simulink model "gm_flash_led"  (R2026a)
settings: Solver=FixedStepDiscrete  StopTime=50
model workspace (MAT data in the model file):
  MAX_COUNT = 5000000
libraries: hdlsllib x2
settings Model: Creator=KoayXianCong  LastModifiedBy=KoayXianCong
settings OptimizationCC: ConditionallyExecuteInputs=off  InheritOutputTypeSmallerThanSingle=on
settings DebuggingCC: ArtificialAlgebraicLoopMsg=error  InheritedTsInSrcMsg=none  SingleTaskRateTransMsg=error
settings HardwareCC: ProdHWDeviceType=ASIC/FPGA->ASIC/FPGA  TargetBitPerPointer=64.0  TargetBitPerSizeT=64.0  TargetBitPerPtrDiffT=64.0  TargetLongLongMode=on  TargetIntDivRoundTo=Zero  TargetEndianess=LittleEndian  TargetWordSize=64.0  TargetHWDeviceType=Custom Processor->MATLAB Host Computer  ProdEqTarget=off

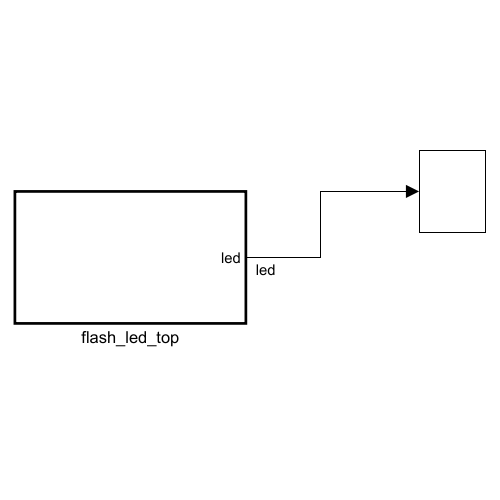
[thumbnail: Simulink's stored preview of the top-level diagram]
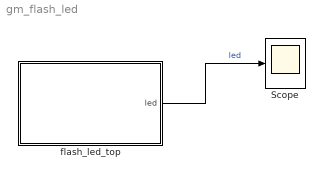
== system gm_flash_led ==
  Scope : Scope
      settings: ActiveDisplayYMinimum=-1  ActiveDisplayYMaximum=1
  flash_led_top : Subsystem  TreatAsAtomicUnit=on
  wires:
  flash_led_top/1(led) -> Scope/1  "led"

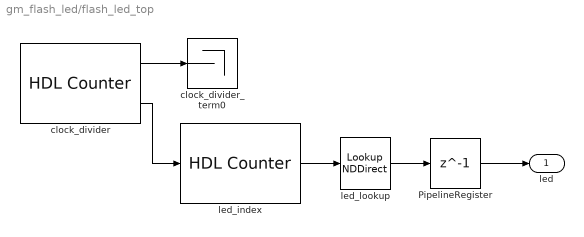
== system gm_flash_led/flash_led_top ==
  PipelineRegister : Delay  DelayLength=1  InitialCondition=0  SampleTime=1
  clock_divider : hdlsllib/Sources/HDL Counter  CountType=Count limited  CountInit=0  CountStep=1  CountMax=MAX_COUNT-1  CountFromType=Initial value  CountFrom=0  CountResetPort=off  CountLoadPort=off  CountEnbPort=off  CountDirPort=off  CountHitOutputPort=on  CountDataType=Unsigned  CountWordLen=23  CountFracLen=0  CountSampTime=1
  clock_divider_term0 : Terminator
  led_index : hdlsllib/Sources/HDL Counter  CountType=Count limited  CountInit=0  CountStep=1  CountMax=7  CountFromType=Initial value  CountFrom=0  CountResetPort=off  CountLoadPort=off  CountEnbPort=on  CountDirPort=off  CountHitOutputPort=off  CountDataType=Unsigned  CountWordLen=3  CountFracLen=0  CountSampTime=1
  led_lookup : LookupNDDirect  NumberOfTableDimensions=1  Table="reshape(uint8([1;2;4;8;16;32;64;128]), [1  8])"  SampleTime=1  TableDataTypeStr=fixdt('uint8')
  led : Outport  SampleTime=1
  wires:
  clock_divider/1 -> clock_divider_term0/1
  clock_divider/2 -> led_index/1
  led_index/1 -> led_lookup/1
  led_lookup/1 -> PipelineRegister/1
  PipelineRegister/1 -> led/1
